simulink model "cic_test1"  (Simulink 6.6)
settings: Solver=FixedStepDiscrete  SolverMode=SingleTasking  StartTime=0.0  StopTime=100  RelTol=1e-3
libraries: dspsigops x7, dspsrcs4 x1
settings Model: Creator=svenhoffmann  LastModifiedBy=svenhoffmann  ExtModeAutoUpdateStatusClock=off
settings OptimizationCC: InlineInvariantSignals=on
settings DebuggingCC: SignalResolutionControl=TryResolveAllWithWarning  MultiTaskDSMMsg=warning  MultiTaskCondExecSysMsg=none  StrictBusMsg=None
settings RTWCC: IncludeERTFirstTime=on

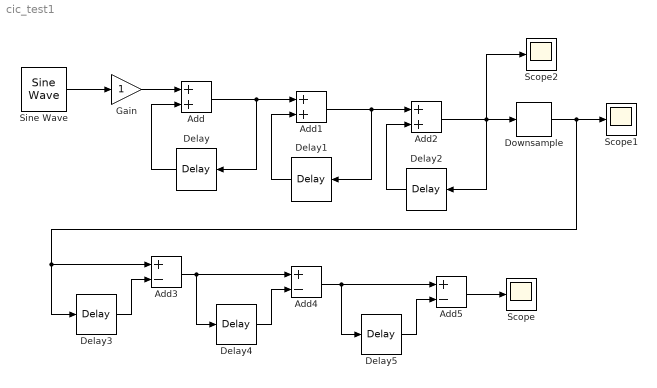
== system cic_test1 ==
  Add : Sum  OutDataTypeMode=int32  OutScaling=2^-10
  Add1 : Sum  OutScaling=2^-10
  Add2 : Sum  OutScaling=2^-10
  Add3 : Sum  Inputs=+-  OutScaling=2^-10
  Add4 : Sum  Inputs=+-  OutScaling=2^-10
  Add5 : Sum  Inputs=+-  OutScaling=2^-10
  Delay : dspsigops/Delay  Orientation=left  dly_unit=Samples  delay=1  ic_detail=off  dif_ic_for_ch=off  dif_ic_for_dly=off  ic=0  reset_popup=None
  Delay1 : dspsigops/Delay  Orientation=left  dly_unit=Samples  delay=1  ic_detail=off  dif_ic_for_ch=off  dif_ic_for_dly=off  ic=0  reset_popup=None
  Delay2 : dspsigops/Delay  Orientation=left  dly_unit=Samples  delay=1  ic_detail=off  dif_ic_for_ch=off  dif_ic_for_dly=off  ic=0  reset_popup=None
  Delay3 : dspsigops/Delay  dly_unit=Samples  delay=1  ic_detail=off  dif_ic_for_ch=off  dif_ic_for_dly=off  ic=0  reset_popup=None
  Delay4 : dspsigops/Delay  dly_unit=Samples  delay=1  ic_detail=off  dif_ic_for_ch=off  dif_ic_for_dly=off  ic=0  reset_popup=None
  Delay5 : dspsigops/Delay  dly_unit=Samples  delay=1  ic_detail=off  dif_ic_for_ch=off  dif_ic_for_dly=off  ic=0  reset_popup=None
  Downsample : dspsigops/Downsample  N=25  phase=0  ic=0  smode=Allow multirate  fmode=Maintain input frame size
  Gain : Gain
  Scope : Scope
      settings: TimeRange=100  YMin=-750000000  YMax=750000000
  Scope1 : Scope
      settings: YMin=-35  YMax=35
  Scope2 : Scope
      settings: YMin=-2.5e+09  YMax=2.5e+09  SaveName=ScopeData2
  Sine Wave : dspsrcs4/Sine Wave  Amplitude=2^15  Frequency=125  Phase=0  SampleMode=Discrete  OutComplex=Real  CompMethod=Table lookup  TableSize=Speed  SampleTime=1/25000  SamplesPerFrame=1  dataType=Fixed-point  wordLen=16  udDataType=sfix()  fracBitsMode=User-defined  numFracBits=0  ResetState=Restart at time zero
  wires:
  Delay/1 -> Add/2
  Add/1 -> Delay/1, Add1/1
  Delay1/1 -> Add1/2
  Add1/1 -> Delay1/1, Add2/1
  Delay2/1 -> Add2/2
  Add2/1 -> Delay2/1, Downsample/1, Scope2/1
  Downsample/1 -> Scope1/1, Add3/1, Delay3/1
  Delay3/1 -> Add3/2
  Delay4/1 -> Add4/2
  Add3/1 -> Add4/1, Delay4/1
  Delay5/1 -> Add5/2
  Add4/1 -> Delay5/1, Add5/1
  Add5/1 -> Scope/1
  Gain/1 -> Add/1
  Sine Wave/1 -> Gain/1
